simulink model "UE03_1d"  (R2022b)
settings: Solver=VariableStepAuto  StartTime=0.0  StopTime=10.0  RelTol=1e-3
settings Model: Creator=basti  LastModifiedBy=basti

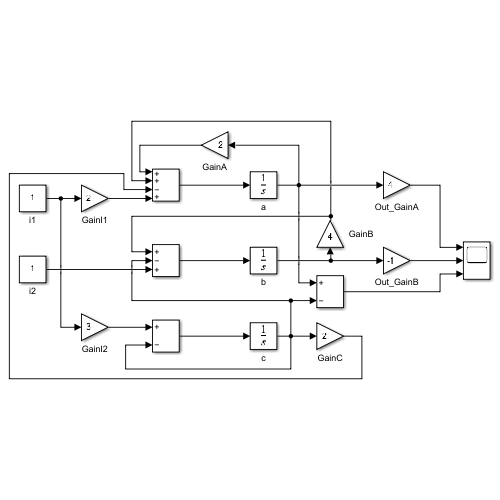
[thumbnail: Simulink's stored preview of the top-level diagram]
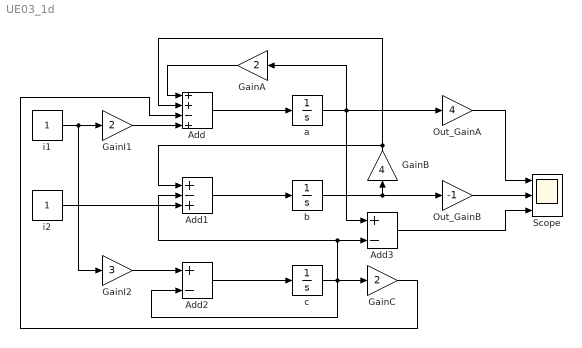
== system UE03_1d ==
  Add : Sum  Inputs=++-+
  Add1 : Sum  Inputs=+-+
  Add2 : Sum  Inputs=+-
  Add3 : Sum  Inputs=+-
  GainA : Gain  Gain=2
  GainB : Gain  Gain=4
  GainC : Gain  Gain=2
  GainI1 : Gain  Gain=2
  GainI2 : Gain  Gain=3
  Out_GainA : Gain  Gain=4
  Out_GainB : Gain  Gain=-1
  Scope : Scope  NumInputPorts=3
  a : Integrator
  b : Integrator
  c : Integrator
  i1 : Constant
  i2 : Constant
  wires:
  i1/1 -> GainI2/1, GainI1/1
  GainI1/1 -> Add/4
  a/1 -> Add3/1, Out_GainA/1, GainA/1
  GainA/1 -> Add/1
  b/1 -> Out_GainB/1, GainB/1
  GainB/1 -> Add1/1, Add/2
  c/1 -> Add3/2, Add1/2, Add2/2, GainC/1
  GainC/1 -> Add/3
  i2/1 -> Add1/3
  GainI2/1 -> Add2/1
  Add/1 -> a/1
  Add1/1 -> b/1
  Add2/1 -> c/1
  Out_GainA/1 -> Scope/1
  Out_GainB/1 -> Scope/2
  Add3/1 -> Scope/3
